simulink library "monroe_library"  (R2012b)
settings: Solver=ode45  StartTime=0.0  StopTime=10.0  RelTol=1e-3
values from neighbouring files (symbols this model uses):
  input_bit_width = ', num2str(input_bit_width))    [fft_direct_draw.m]
undefined symbols (not defined in the file or in its folder): gcbh, xlBlockLoadCallback
libraries: xbsIndex_r4 x1880, monroe_library x159, casper_library x13, xps_library x1
(part 21 of 43)

== system monroe_library/direct_coeff_gen/coeff_gen_stage_2_group_4 ==
  sync : Inport
  Concat : xbsIndex_r4/Concat  num_inputs=2  dbl_ovrd=off  block_type=concat
  Concat1 : xbsIndex_r4/Concat  num_inputs=2  dbl_ovrd=off  block_type=concat
  Concat2 : xbsIndex_r4/Concat  num_inputs=2  dbl_ovrd=off  block_type=concat
  Constant : xbsIndex_r4/Constant  arith_type=Boolean  const=0  n_bits=16  bin_pt=14  explicit_period=on  period=1  equ=P=C  opselect=C  inp2=PCIN>>17  opr=+  inp1=P  carry=CIN  dbl_ovrd=off  block_type=constant
  Constant1 : xbsIndex_r4/Constant  arith_type=Boolean  const=1  n_bits=16  bin_pt=14  explicit_period=off  period=1  equ=P=C  opselect=C  inp2=PCIN>>17  opr=+  inp1=P  carry=CIN  dbl_ovrd=off  block_type=constant
  Constant3 : xbsIndex_r4/Constant  arith_type=Signed (2's comp)  const=0  n_bits=18  bin_pt=17  explicit_period=on  period=1  equ=P=C  opselect=C  inp2=PCIN>>17  opr=+  inp1=P  carry=CIN  dbl_ovrd=off  block_type=constant
  Constant4 : xbsIndex_r4/Constant  arith_type=Boolean  const=0  n_bits=16  bin_pt=14  explicit_period=off  period=1  equ=P=C  opselect=C  inp2=PCIN>>17  opr=+  inp1=P  carry=CIN  dbl_ovrd=off  block_type=constant
  Constant5 : xbsIndex_r4/Constant  arith_type=Unsigned  const=2  n_bits=10  bin_pt=0  explicit_period=on  period=1  equ=P=C  opselect=C  inp2=PCIN>>17  opr=+  inp1=P  carry=CIN  dbl_ovrd=off  block_type=constant
  Counter : xbsIndex_r4/Counter  cnt_type=Free Running  cnt_to=Inf  operation=Up  start_count=0  cnt_by_val=1  arith_type=Unsigned  n_bits=10  bin_pt=0  load_pin=on  rst=off  en=off  explicit_period=on  period=1  dbl_ovrd=off  use_behavioral_HDL=off  implementation=Fabric  block_type=counter
  Delay : xbsIndex_r4/Delay  en=off  latency=0  dbl_ovrd=off  reg_retiming=off  block_type=delay
  Dual Port RAM4 : xbsIndex_r4/Dual Port RAM  depth=2048  initVector=[-1 -0.999998823451702 -0.999995293809576 -0.999989411081928 -0.999981175282601 -0.999970586430974 -0.999957644551964 -0.999942349676024 -0.999924701839145 -0.999904701082853 -0.999882347454213 -0.999857641005824 -0.999830581795823 -0.999801169887884 -0.999769405351215 -0.999735288260562 -0.999698818696204 -0.999659996743959 -0.999618822495179 -0.999575296046749 -0.999529417501093 -0.999481186966167 -0.999430604555462 -0.999377670388003 -0.99932238458835 -0.999264747286594 -0.999204758618364 -0.999142418724817 -0.999077727752645 -0.999010685854073 -0.998941293186857 -0.998869549914284 -0.998795456205172 -0.998719012233873 -0.998640218180265 -0.998559074229759 -0.998475580573295 -0.99838973740734 -0.998301544933893 -0.998211003360478 -0.998118112900149 -0.998022873771486 -0.997925286198596 -0.997825350411112 -0.997723066644192 -0.99761843513852 -0.997511456140303 -0.997402129901275 -0.99729045667869 -0.997176436735326 -0.997060070339483 -0.996941357764982 -0.996820299291166 -0.996696895202896 -0.996571145790555 -0.996443051350043 -0.996312612182778 -0.996179828595697 -0.996044700901252 -0.995907229417412 -0.99576741446766 -0.995625256380994 -0.995480755491927 -0.995333912140482 -0.995184726672197 -0.995033199438119 -0.994879330794806 -0.994723121104326 -0.994564570734255 -0.994403680057679 -0.994240449453188 -0.994074879304879 -0.993906970002356 -0.993736721940725 -0.993564135520595 -0.993389211148081 -0.993211949234795 -0.993032350197851 -0.992850414459865 -0.992666142448948 -0.99247953459871 -0.992290591348257 -0.992099313142192 -0.991905700430609 -0.9917097536691 -0.991511473318744 -0.991310859846115 -0.991107913723277 -0.99090263542778 -0.990695025442665 -0.990485084256457 -0.990272812363169 -0.990058210262297 -0.989841278458821 -0.989622017463201 -0.98940042779138 -0.989176509964781 -0.988950264510303 -0.988721691960324 -0.988490792852697 -0.988257567730749 -0.988022017143284 -0.987784141644572 -0.987543941794359 -0.987301418157858 -0.987056571305751 -0.986809401814186 -0.986559910264776 -0.986308097244599 -0.986053963346195 -0.985797509167567 -0.985538735312176 -0.985277642388941 -0.98501423101224 -0.984748501801904 -0.984480455383221 -0.984210092386929 -0.983937413449219 -0.98366241921173 -0.983385110321551 -0.983105487431216 -0.982823551198705 -0.982539302287441 -0.982252741366289 -0.981963869109555 -0.981672686196983 -0.981379193313755 -0.981083391150487 -0.98078528040323 -0.980484861773469 -0.980182135968117 -0.979877103699518 -0.979569765685441 -0.979260122649082 -0.978948175319062 -0.978633924429423 -0.978317370719628 -0.977998514934557 -0.97767735782451 -0.9773539001452 -0.977028142657754 -0.976700086128712 -0.976369731330021 -0.976037079039039 -0.975702130038529 -0.975364885116657 -0.975025345066994 -0.974683510688511 -0.974339382785576 -0.973992962167956 -0.973644249650812 -0.973293246054698 -0.97293995220556 -0.972584368934732 -0.972226497078936 -0.971866337480279 -0.971503890986252 -0.971139158449725 -0.97077214072895 -0.970402838687556 -0.970031253194544 -0.969657385124292 -0.969281235356549 -0.968902804776429 -0.968522094274417 -0.968139104746362 -0.967753837093476 -0.967366292222329 -0.966976471044852 -0.966584374478333 -0.966190003445413 -0.965793358874084 -0.965394441697689 -0.96499325285492 -0.964589793289813 -0.964184063951746 -0.96377606579544 -0.963365799780954 -0.962953266873684 -0.962538468044359 -0.962121404269042 -0.961702076529123 -0.961280485811321 -0.96085663310768 -0.960430519415566 -0.960002145737666 -0.959571513081985 -0.959138622461842 -0.958703474895872 -0.958266071408018 -0.957826413027533 -0.957384500788976 -0.956940335732209 -0.956493918902395 -0.956045251349997 -0.955594334130771 -0.955141168305771 -0.954685754941338 -0.954228095109106 -0.95376818988599 -0.953306040354194 -0.952841647601199 -0.952375012719766 -0.951906136807932 -0.951435020969008 -0.950961666311575 -0.950486073949482 -0.950008245001843 -0.949528180593037 -0.949045881852701 -0.94856134991573 -0.948074585922276 ...(+34800 chars)]  distributed_mem=Block RAM  init_a=0  init_b=0  rst_a=off  rst_b=off  en_a=off  en_b=off  latency=2  write_mode_A=No Read On Write  write_mode_B=No Read On Write  dbl_ovrd=off  optimize=Area  use_rpm=on  block_type=dpram
  Reinterpret : xbsIndex_r4/Reinterpret  force_arith_type=on  arith_type=Unsigned  force_bin_pt=on  bin_pt=0  block_type=reinterpret
      settings: infoedit="Changes signal type without altering the binary representation.   You can changed the signal between signed and unsigned, and relocate the binary point.<br><br>Hardware notes: In hardware this block costs nothing.<br><br>Example:  Suppose the input is 6 bits wide, signed, with 2 fractional bits, and the output is forced to unsigned with 0 fractional bits.  Then an input of -2.0 (1110.00 in binary 2's complement) becomes an output of 56 (111000 in binary)."
  Reinterpret1 : xbsIndex_r4/Reinterpret  force_arith_type=on  arith_type=Unsigned  force_bin_pt=on  bin_pt=0  block_type=reinterpret
      settings: infoedit="Changes signal type without altering the binary representation.   You can changed the signal between signed and unsigned, and relocate the binary point.<br><br>Hardware notes: In hardware this block costs nothing.<br><br>Example:  Suppose the input is 6 bits wide, signed, with 2 fractional bits, and the output is forced to unsigned with 0 fractional bits.  Then an input of -2.0 (1110.00 in binary 2's complement) becomes an output of 56 (111000 in binary)."
  count_slice : xbsIndex_r4/Slice  nbits=10  boolean_output=off  mode=Upper Bit Location + Width  bit1=0  base1=MSB of Input  bit0=0  base0=MSB of Input  dbl_ovrd=off  block_type=slice
  coeff : Outport
  wires:
  count_slice/1 -> Concat1/2, Concat/2  "xlsub2_Counter_out1"
  Constant3/1 -> Dual Port RAM4/5, Dual Port RAM4/2  "xlsub2_Constant3_out1"
  Constant/1 -> Dual Port RAM4/6, Dual Port RAM4/3  "xlsub2_Constant_out1"
  Reinterpret1/1 -> Concat2/2  "xlsub2_Reinterpret1_out1"
  Dual Port RAM4/2 -> Reinterpret1/1  "xlsub2_Dual_Port_RAM4_out2"
  Reinterpret/1 -> Concat2/1  "xlsub2_Reinterpret_out1"
  Dual Port RAM4/1 -> Reinterpret/1  "xlsub2_Dual_Port_RAM4_out1"
  Concat1/1 -> Dual Port RAM4/4  "xlsub2_Concat1_out1"
  Concat/1 -> Dual Port RAM4/1  "xlsub2_Concat_out1"
  Delay/1 -> coeff/1
  Concat2/1 -> Delay/1  "xlsub2_Concat2_out1"
  Counter/1 -> count_slice/1
  Constant5/1 -> Counter/2  "xlsub2_Constant5_out1"
  sync/1 -> Counter/1
  Constant4/1 -> Concat1/1  "xlsub2_Constant4_out1"
  Constant1/1 -> Concat/1  "xlsub2_Constant1_out1"
